simulink model "EV_Modeling_old"  (R2024b)
settings: Solver=FixedStepAuto  StartTime=0.0  StopTime=10382  FixedStep=0.1  RelTol=1e-3
values from neighbouring files (symbols this model uses):
  battery_SOC_SOC = battery_SOC(:,1)    [EV_Truck.m]    (also in simulink.m)
  battery_SOC_voltage = battery_SOC(:,2)    [EV_Truck.m]    (also in simulink.m)
  drag_coefficient_FV1 = table2array(drag_coefficient(:,3))    [simulink.m]
  drag_coefficient_FV2 = table2array(drag_coefficient(:,4))    [simulink.m]
  drag_coefficient_input = table2array(drag_coefficient(:,1))    [simulink.m]
  drag_coefficient_LV = table2array(drag_coefficient(:,2))    [simulink.m]
  electric_consumption_ressistancce = electric_consumption(:,2)    [EV_Truck.m]    (also in simulink.m)
  electric_consumption_voltage = electric_consumption(:,1)    [EV_Truck.m]    (also in simulink.m)
  motor_efficiency_efficiency = table2array(motor_efficiency(2:height(motor_efficiency),2:width(motor_efficiency)))    [EV_Truck.m]    (also in simulink.m)
  motor_efficiency_RPM = table2array(motor_efficiency(2:height(motor_efficiency),1))    [EV_Truck.m]    (also in simulink.m)
  motor_efficiency_torque = transpose(motor_efficiency_torque)    [EV_Truck.m]    (also in simulink.m)
  motor_RPM_torque = table2array(motor_torque(1:14,1))    [EV_Truck.m]    (also in simulink.m)
  motor_torque_RPM = table2array(motor_torque(1:14,2))    [EV_Truck.m]    (also in simulink.m)
undefined symbols (not defined in the file or in its folder): battery_builder_rtmsupport, battery_sli_rtmsupport, C1_mat, C2_mat, c_sqrt, DiscIntNeverNeededParam, dV0_mat, gcbh, n, Wc, Wm, x0
libraries: simulink x87, packLibrary_lib x30, nesl_utility x6, fl_lib x6, simulink_extras x3, mpcadaslib x2, slpidlib x1
(part 8 of 12)

== system EV_Modeling_old/FV1/SOC Estimator (Kalman Filter)1/Kalman Filter/EKF/Delay - X ==
  u : Inport
  SOC0 : Inport  Port=2
  Constant1 : Constant  Value=0  OutDataTypeStr=Inherit: Inherit via back propagation
  Data Type Conversion Inherited : simulink/Signal Attributes/Data Type Conversion Inherited  ConvertRealWorld=Real World Value  DoSatur=off
  Delay : Delay  DelayLength=1  InitialConditionSource=Input port  SampleTime=Ts
      settings: InputPortMap=u0,p4
  Mux : Mux  Inputs=2
  y : Outport
  wires:
  SOC0/1 -> Data Type Conversion Inherited/1, Mux/1
  Mux/1 -> Delay/2
  Delay/1 -> y/1
  u/1 -> Delay/1
  Data Type Conversion Inherited/1 -> Mux/2
  Constant1/1 -> Data Type Conversion Inherited/2

== system EV_Modeling_old/FV1/SOC Estimator (Kalman Filter)1/Kalman Filter/EKF/Jacobian ==
  current : Inport
  Temperature : Inport  Port=2
  x : Inport  Port=3
  -Ts : Gain  Gain=-1
  2-D Lookup Table C1 : Lookup_n-D  NumberOfTableDimensions=1  BreakpointsForDimension1=SOC_vec  BreakpointsForDimension2=T_vec  Table=C1_mat  InternalRulePriority=Speed  RndMeth=Simplest
  2-D Lookup Table R0 : Lookup_n-D  NumberOfTableDimensions=1  BreakpointsForDimension1=SOC_vec  BreakpointsForDimension2=T_vec  Table=R0_mat  InternalRulePriority=Speed  RndMeth=Simplest
  2-D Lookup Table R1 : Lookup_n-D  NumberOfTableDimensions=1  BreakpointsForDimension1=SOC_vec  BreakpointsForDimension2=T_vec  Table=R1_mat  InternalRulePriority=Speed  RndMeth=Simplest
  2-D Lookup Table V0 : Lookup_n-D  NumberOfTableDimensions=1  BreakpointsForDimension1=SOC_vec  BreakpointsForDimension2=T_vec  Table=V0_mat  InternalRulePriority=Speed  RndMeth=Simplest
  2-D Lookup Table dV0 : Lookup_n-D  NumberOfTableDimensions=1  BreakpointsForDimension1=SOC_vec  BreakpointsForDimension2=T_vec  Table=dV0_mat  InternalRulePriority=Speed  RndMeth=Simplest
  Assignment : Assignment  NumberOfDimensions=2  DiagnosticForDimensions=Warning  IndexOptions=Index vector (dialog),Index vector (dialog)  Indices=2,2  OutputSizes=1,1
  Constant : Constant  Value=|  OutDataTypeStr=Inherit: Inherit via back propagation
      | [1 0;
      | 0 0]
  Constant1 : Constant  OutDataTypeStr=Inherit: Inherit via back propagation
  Constant4 : Constant  Value=-1  OutDataTypeStr=Inherit: Inherit via back propagation
  Data Type Conversion Inherited : simulink/Signal Attributes/Data Type Conversion Inherited  ConvertRealWorld=Real World Value  DoSatur=off
  Data Type Conversion Inherited1 : simulink/Signal Attributes/Data Type Conversion Inherited  ConvertRealWorld=Real World Value  DoSatur=off
  Data Type Conversion Inherited2 : simulink/Signal Attributes/Data Type Conversion Inherited  ConvertRealWorld=Real World Value  DoSatur=off
  Gain : Gain  Gain=1/(AH*3600)
  Math Function : Math
  Mux : Mux  Inputs=2
  Mux1 : Mux  Inputs=2
  Probe : Probe  ProbeWidth=off  ProbeComplexSignal=off  ProbeSampleTimeDataType=Same as input
  Product : Product
  Product2 : Product  Inputs=/*
  Product4 : Product
  Product6 : Product
  Selector : Selector  InputPortWidth=2  IndexOptions=Index vector (dialog)  Indices=1  OutputSizes=1
  Selector1 : Selector  InputPortWidth=2  IndexOptions=Index vector (dialog)  Indices=2  OutputSizes=1
  Selector2 : Selector  InputPortWidth=2  IndexOptions=Index vector (dialog)  Indices=1  OutputSizes=1
  Sum : Sum  Inputs=-+|
  Sum2 : Sum  Inputs=+--
  Terminator : Terminator
  Transpose1 : Math  Operator=transpose
  Vt_model : Outport
  H : Outport  Port=2
  F : Outport  Port=3
  G : Outport  Port=4
  wires:
  Gain/1 -> Mux/1
  Selector/1 -> 2-D Lookup Table R1/1, 2-D Lookup Table R0/1, 2-D Lookup Table V0/1, 2-D Lookup Table dV0/1, 2-D Lookup Table C1/1  "SOC"
  x/1 -> Probe/1, Selector/1, Selector1/1
  Math Function/1 -> Sum/1, Assignment/2
  2-D Lookup Table R1/1 -> Product4/2, Product/1  "R1"
  2-D Lookup Table C1/1 -> Product/2  "C1"
  Product2/1 -> Math Function/1
  Assignment/1 -> F/1
  Sum/1 -> Product4/1
  -Ts/1 -> Data Type Conversion Inherited/1, Data Type Conversion Inherited1/1, Gain/1, Product2/2
  Product4/1 -> Mux/2
  Mux/1 -> G/1
  2-D Lookup Table R0/1 -> Product6/1  "R0"
  Product6/1 -> Sum2/2
  Selector1/1 -> Sum2/3  "V1"
  current/1 -> Product6/2
  Mux1/1 -> Transpose1/1
  Transpose1/1 -> H/1
  Sum2/1 -> Vt_model/1
  2-D Lookup Table V0/1 -> Sum2/1  "V0"
  2-D Lookup Table dV0/1 -> Data Type Conversion Inherited2/1, Mux1/1  "dV0"
  Product/1 -> Product2/1  "tau1"
  Probe/1 -> Selector2/1
  Selector2/1 -> -Ts/1
  Data Type Conversion Inherited/1 -> Assignment/1
  Constant/1 -> Data Type Conversion Inherited/2
  Data Type Conversion Inherited1/1 -> Sum/2
  Constant1/1 -> Data Type Conversion Inherited1/2
  Data Type Conversion Inherited2/1 -> Mux1/2
  Constant4/1 -> Data Type Conversion Inherited2/2
  Temperature/1 -> Terminator/1

== system EV_Modeling_old/FV1/SOC Estimator (Kalman Filter)1/Kalman Filter/EKF/Prediction ==
  F : Inport
  G : Inport  Port=2
  xk_k : Inport  Port=3
  Pk_k : Inport  Port=4
  Current : Inport  Port=5
  Constant : Constant  Value=Q  OutDataTypeStr=Inherit: Inherit via back propagation
  Product : Product  Multiplication=Matrix(*)
  Product1 : Product  Multiplication=Matrix(*)
  Product2 : Product  Inputs=3  Multiplication=Matrix(*)
  Sum : Sum  Inputs=|++
  Sum1 : Sum  Inputs=|++
  Transpose : Math  Operator=transpose
  xk1_k : Outport
  Pk1_k : Outport  Port=2
  wires:
  F/1 -> Transpose/1, Product2/1, Product/1
  xk_k/1 -> Product/2
  G/1 -> Product1/1
  Current/1 -> Product1/2
  Product/1 -> Sum/1
  Product1/1 -> Sum/2
  Sum/1 -> xk1_k/1
  Pk_k/1 -> Product2/2
  Transpose/1 -> Product2/3
  Product2/1 -> Sum1/1
  Sum1/1 -> Pk1_k/1
  Constant/1 -> Sum1/2

== system EV_Modeling_old/FV1/SOC Estimator (Kalman Filter)1/Kalman Filter/EKF 2RC/Correction ==
  Vt_error : Inport
  H : Inport  Port=2
  xk1_k : Inport  Port=3
  Pk1_k : Inport  Port=4
  Constant : Constant  Value=R
  Constant1 : Constant  Value=eye(size(R,1))
  Constant2 : Constant  Value=eye(size(Q_2RC,1))
  Data Type Conversion Inherited : simulink/Signal Attributes/Data Type Conversion Inherited  ConvertRealWorld=Real World Value  DoSatur=off
  Data Type Conversion Inherited1 : simulink/Signal Attributes/Data Type Conversion Inherited  ConvertRealWorld=Real World Value  DoSatur=off
  Data Type Conversion Inherited2 : simulink/Signal Attributes/Data Type Conversion Inherited  ConvertRealWorld=Real World Value  DoSatur=off
  Divide : Product  Inputs=*/  Multiplication=Matrix(*)
  Product{,1,3..5} (5 alike) : Product  Multiplication=Matrix(*)
  Product2 : Product  Inputs=3  Multiplication=Matrix(*)
  Sum : Sum  Inputs=++|
  Sum2 : Sum  Inputs=|++
  Sum3 : Sum  Inputs=-+|
  Transpose : Math  Operator=transpose
  xk1_k1 : Outport
  Pk1_k1 : Outport  Port=2
  wires:
  Constant2/1 -> Data Type Conversion Inherited2/2
  Data Type Conversion Inherited2/1 -> Sum3/2
  Constant1/1 -> Data Type Conversion Inherited1/2
  Data Type Conversion Inherited1/1 -> Divide/1
  Constant/1 -> Data Type Conversion Inherited/2
  Data Type Conversion Inherited/1 -> Sum2/2
  H/1 -> Product4/2, Data Type Conversion Inherited2/1, Product2/1, Transpose/1
  Transpose/1 -> Product2/3, Product/2
  Pk1_k/1 -> Product5/2, Product2/2, Product/1
  Product/1 -> Product1/1, Data Type Conversion Inherited1/1
  Product2/1 -> Sum2/1, Data Type Conversion Inherited/1
  Product1/1 -> Product4/1, Product3/1  "Kk1"
  Sum2/1 -> Divide/2
  Divide/1 -> Product1/2
  xk1_k/1 -> Sum/2
  Vt_error/1 -> Product3/2
  Product3/1 -> Sum/1
  Sum/1 -> xk1_k1/1
  Product4/1 -> Sum3/1
  Sum3/1 -> Product5/1
  Product5/1 -> Pk1_k1/1

== system EV_Modeling_old/FV1/SOC Estimator (Kalman Filter)1/Kalman Filter/EKF 2RC/Delay - X ==
  u : Inport
  SOC0 : Inport  Port=2
  Constant1 : Constant  Value=0
  Data Type Conversion Inherited : simulink/Signal Attributes/Data Type Conversion Inherited  ConvertRealWorld=Real World Value  DoSatur=off
  Delay : Delay  DelayLength=1  InitialConditionSource=Input port  SampleTime=Ts
      settings: InputPortMap=u0,p4
  Mux : Mux  Inputs=3
  y : Outport
  wires:
  Constant1/1 -> Data Type Conversion Inherited/2
  Data Type Conversion Inherited/1 -> Mux/3, Mux/2
  SOC0/1 -> Mux/1, Data Type Conversion Inherited/1
  Mux/1 -> Delay/2
  Delay/1 -> y/1
  u/1 -> Delay/1

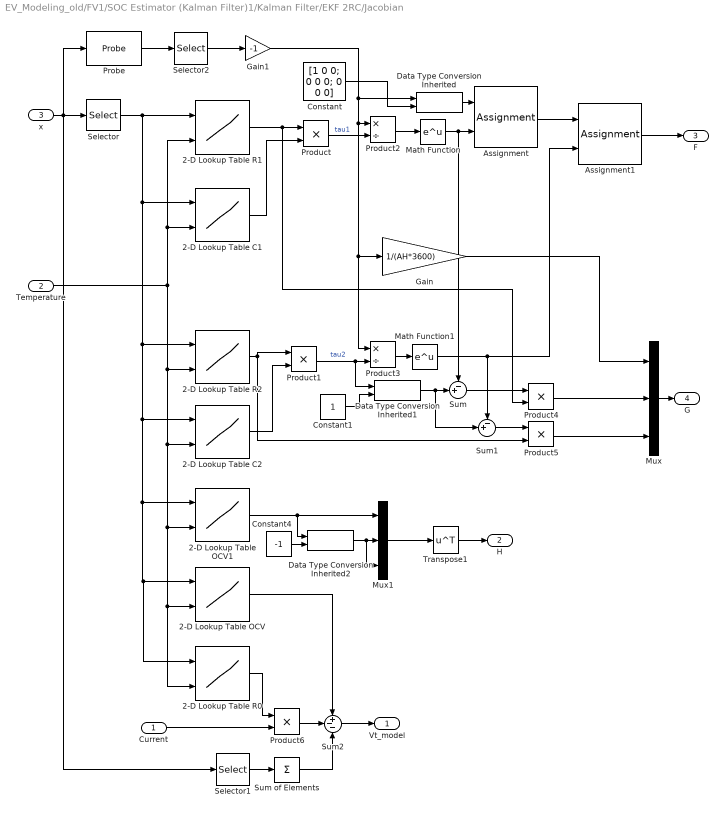
== system EV_Modeling_old/FV1/SOC Estimator (Kalman Filter)1/Kalman Filter/EKF 2RC/Jacobian ==
  Current : Inport
  Temperature : Inport  Port=2
  x : Inport  Port=3
  2-D Lookup Table C1 : Lookup_n-D  BreakpointsForDimension1=SOC_vec  BreakpointsForDimension2=T_vec  Table=C1_mat  InternalRulePriority=Speed  RndMeth=Simplest
      settings: InputPortMap=u0,u1
  2-D Lookup Table C2 : Lookup_n-D  BreakpointsForDimension1=SOC_vec  BreakpointsForDimension2=T_vec  Table=C2_mat  InternalRulePriority=Speed  RndMeth=Simplest
      settings: InputPortMap=u0,u1
  2-D Lookup Table OCV : Lookup_n-D  BreakpointsForDimension1=SOC_vec  BreakpointsForDimension2=T_vec  Table=V0_mat  InternalRulePriority=Speed  RndMeth=Simplest
      settings: InputPortMap=u0,u1
  2-D Lookup Table OCV1 : Lookup_n-D  BreakpointsForDimension1=SOC_vec  BreakpointsForDimension2=T_vec  Table=dV0_mat  InternalRulePriority=Speed  RndMeth=Simplest
      settings: InputPortMap=u0,u1
  2-D Lookup Table R0 : Lookup_n-D  BreakpointsForDimension1=SOC_vec  BreakpointsForDimension2=T_vec  Table=R0_mat  InternalRulePriority=Speed  RndMeth=Simplest
      settings: InputPortMap=u0,u1
  2-D Lookup Table R1 : Lookup_n-D  BreakpointsForDimension1=SOC_vec  BreakpointsForDimension2=T_vec  Table=R1_mat  InternalRulePriority=Speed  RndMeth=Simplest
      settings: InputPortMap=u0,u1
  2-D Lookup Table R2 : Lookup_n-D  BreakpointsForDimension1=SOC_vec  BreakpointsForDimension2=T_vec  Table=R2_mat  InternalRulePriority=Speed  RndMeth=Simplest
      settings: InputPortMap=u0,u1
  Assignment : Assignment  NumberOfDimensions=2  DiagnosticForDimensions=Warning  IndexOptions=Index vector (dialog),Index vector (dialog)  Indices=2,2  OutputSizes=1,1
  Assignment1 : Assignment  NumberOfDimensions=2  DiagnosticForDimensions=Warning  IndexOptions=Index vector (dialog),Index vector (dialog)  Indices=3,3  OutputSizes=1,1
  Constant : Constant  Value=|
      | [1 0  0;
      | 0 0 0;
      | 0 0 0]
  Constant1 : Constant
  Constant4 : Constant  Value=-1
  Data Type Conversion Inherited : simulink/Signal Attributes/Data Type Conversion Inherited  ConvertRealWorld=Real World Value  DoSatur=off
  Data Type Conversion Inherited1 : simulink/Signal Attributes/Data Type Conversion Inherited  ConvertRealWorld=Real World Value  DoSatur=off
  Data Type Conversion Inherited2 : simulink/Signal Attributes/Data Type Conversion Inherited  ConvertRealWorld=Real World Value  DoSatur=off
  Gain : Gain  Gain=1/(AH*3600)
  Gain1 : Gain  Gain=-1
  Math Function : Math
  Math Function1 : Math
  Mux : Mux  Inputs=3
  Mux1 : Mux  Inputs=3
  Probe : Probe  ProbeWidth=off  ProbeComplexSignal=off  ProbeSampleTimeDataType=Same as input
  Product{,1,4..6} (5 alike) : Product
  Product2 : Product  Inputs=*/
  Product3 : Product  Inputs=*/
  Selector : Selector  InputPortWidth=3  IndexOptions=Index vector (dialog)  Indices=1  OutputSizes=1
  Selector1 : Selector  InputPortWidth=3  IndexOptions=Index vector (dialog)  Indices=[2 3]  OutputSizes=1
  Selector2 : Selector  InputPortWidth=2  IndexOptions=Index vector (dialog)  Indices=1  OutputSizes=1
  Sum : Sum  Inputs=-+|
  Sum of Elements : Sum  Inputs=+
  Sum1 : Sum  Inputs=-+|
  Sum2 : Sum  Inputs=+--
  Transpose1 : Math  Operator=transpose
  Vt_model : Outport
  H : Outport  Port=2
  F : Outport  Port=3
  G : Outport  Port=4
  wires:
  Data Type Conversion Inherited2/1 -> Mux1/2, Mux1/3
  Constant4/1 -> Data Type Conversion Inherited2/2
  Constant1/1 -> Data Type Conversion Inherited1/2
  Data Type Conversion Inherited1/1 -> Sum/2, Sum1/2
  Constant/1 -> Data Type Conversion Inherited/2
  Data Type Conversion Inherited/1 -> Assignment/1
  x/1 -> Probe/1, Selector1/1, Selector/1
  Assignment/1 -> Assignment1/1
  Math Function1/1 -> Sum1/1, Assignment1/2
  Math Function/1 -> Assignment/2, Sum/1
  2-D Lookup Table R1/1 -> Product4/2, Product/1
  2-D Lookup Table C1/1 -> Product/2
  2-D Lookup Table R2/1 -> Product1/1, Product5/2
  2-D Lookup Table C2/1 -> Product1/2
  Product/1 -> Product2/2  "tau1"
  Product1/1 -> Product3/2, Data Type Conversion Inherited1/1  "tau2"
  Product2/1 -> Math Function/1
  Product3/1 -> Math Function1/1
  Assignment1/1 -> F/1
  Sum/1 -> Product4/1
  Sum1/1 -> Product5/1
  Gain1/1 -> Product3/1, Gain/1, Product2/1, Data Type Conversion Inherited/1
  Product4/1 -> Mux/2
  Product5/1 -> Mux/3
  Mux/1 -> G/1
  2-D Lookup Table R0/1 -> Product6/1
  Product6/1 -> Sum2/2
  Selector1/1 -> Sum of Elements/1
  Sum of Elements/1 -> Sum2/3
  Current/1 -> Product6/2
  Mux1/1 -> Transpose1/1
  Transpose1/1 -> H/1
  Sum2/1 -> Vt_model/1
  2-D Lookup Table OCV/1 -> Sum2/1
  2-D Lookup Table OCV1/1 -> Mux1/1, Data Type Conversion Inherited2/1
  Temperature/1 -> 2-D Lookup Table R1/2, 2-D Lookup Table C1/2, 2-D Lookup Table R0/2, 2-D Lookup Table OCV/2, 2-D Lookup Table OCV1/2, 2-D Lookup Table C2/2, 2-D Lookup Table R2/2
  Selector/1 -> 2-D Lookup Table R0/1, 2-D Lookup Table OCV/1, 2-D Lookup Table OCV1/1, 2-D Lookup Table C2/1, 2-D Lookup Table R2/1, 2-D Lookup Table C1/1, 2-D Lookup Table R1/1
  Gain/1 -> Mux/1
  Probe/1 -> Selector2/1
  Selector2/1 -> Gain1/1

== system EV_Modeling_old/FV1/SOC Estimator (Kalman Filter)1/Kalman Filter/EKF 2RC/Prediction ==
  F : Inport
  G : Inport  Port=2
  xk_k : Inport  Port=3
  Pk_k : Inport  Port=4
  Current : Inport  Port=5
  Constant : Constant  Value=Q_2RC
  Data Type Conversion Inherited : simulink/Signal Attributes/Data Type Conversion Inherited  ConvertRealWorld=Real World Value  DoSatur=off
  Product : Product  Multiplication=Matrix(*)
  Product1 : Product  Multiplication=Matrix(*)
  Product2 : Product  Inputs=3  Multiplication=Matrix(*)
  Sum : Sum  Inputs=|++
  Sum1 : Sum  Inputs=|++
  Transpose : Math  Operator=transpose
  xk1_k : Outport
  Pk1_k : Outport  Port=2
  wires:
  Constant/1 -> Data Type Conversion Inherited/2
  Data Type Conversion Inherited/1 -> Sum1/2
  F/1 -> Transpose/1, Data Type Conversion Inherited/1, Product2/1, Product/1
  xk_k/1 -> Product/2
  G/1 -> Product1/1
  Current/1 -> Product1/2
  Product/1 -> Sum/1
  Product1/1 -> Sum/2
  Sum/1 -> xk1_k/1
  Pk_k/1 -> Product2/2
  Transpose/1 -> Product2/3
  Product2/1 -> Sum1/1
  Sum1/1 -> Pk1_k/1

== system EV_Modeling_old/FV1/SOC Estimator (Kalman Filter)1/Kalman Filter/UKBF/Prediction-correction ==
  Current : Inport
  Temperature : Inport  Port=2
  Voltage : Inport  Port=3
  X0 : Inport  Port=4
  Integrator1 : Integrator  InitialConditionSource=external
  Measurement function : Subsystem  TreatAsAtomicUnit=on
  State function : Subsystem  TreatAsAtomicUnit=on
  Sum of Elements1 : Sum  Inputs=+  CollapseMode=Specified dimension  CollapseDim=2
  Sum of Elements2 : Sum  Inputs=+  CollapseMode=Specified dimension  CollapseDim=2
  Sum of Elements3 : Sum  Inputs=+  CollapseMode=Specified dimension  CollapseDim=2
  Update A : Subsystem
  Xdot : Subsystem
  xhat : Outport
  wires:
  Integrator1/1 -> State function/3(X), Measurement function/3(X), Xdot/7(X), Update A/1(X)
  Voltage/1 -> Xdot/1(Voltage)
  Measurement function/1(h(X)) -> Xdot/2(h(X))
  State function/1(f(X)) -> Xdot/4(f(X))
  X0/1 -> Integrator1/2
  Current/1 -> State function/1(Current), Measurement function/1(Current)
  Temperature/1 -> State function/2(Temperature), Measurement function/2(Temperature)
  Update A/2(xhat) -> xhat/1
  Update A/1(A(t)) -> Xdot/8(A)
  Xdot/1(Xdot) -> Integrator1/1
  Measurement function/2(h(X)*Wm) -> Sum of Elements1/1
  State function/2(f(X)*Wm) -> Sum of Elements2/1
  State function/3(X*Wm) -> Sum of Elements3/1
  Sum of Elements1/1 -> Xdot/3(mh)
  Sum of Elements2/1 -> Xdot/5(mf)
  Sum of Elements3/1 -> Xdot/6(mx)

== system EV_Modeling_old/FV1/SOC Estimator (Kalman Filter)1/Kalman Filter/UKBF/Sigma points init ==
  x0 : Inport
  A : Inport  Port=2
  Assignment : Assignment  NumberOfDimensions=2  DiagnosticForDimensions=Warning  IndexOptions=Index vector (dialog),Index vector (dialog)  Indices=1:n,1  OutputSizes=1,1
  Assignment1 : Assignment  NumberOfDimensions=2  DiagnosticForDimensions=Warning  IndexOptions=Index vector (dialog),Index vector (dialog)  Indices=1:n,2:n+1  OutputSizes=1,1
  Assignment2 : Assignment  NumberOfDimensions=2  DiagnosticForDimensions=Warning  IndexOptions=Index vector (dialog),Index vector (dialog)  Indices=1:n,n+2:2*n+1  OutputSizes=1,1
  Constant : Constant  Value=zeros(n,2*n+1)
  Constant1 : Constant  Value=ones(1,n)  VectorParams1D=off
  Gain : Gain  Gain=c_sqrt
  Matrix Multiply : Product  Multiplication=Matrix(*)
  Sum : Sum  Inputs=|++
  Sum1 : Sum  Inputs=|+-
  X0 : Outport
  wires:
  A/1 -> Gain/1
  x0/1 -> Matrix Multiply/1, Assignment/2
  Constant1/1 -> Matrix Multiply/2
  Matrix Multiply/1 -> Sum1/1, Sum/1
  Gain/1 -> Sum1/2, Sum/2
  Sum/1 -> Assignment1/2
  Sum1/1 -> Assignment2/2
  Constant/1 -> Assignment/1
  Assignment/1 -> Assignment1/1
  Assignment1/1 -> Assignment2/1
  Assignment2/1 -> X0/1

== system EV_Modeling_old/FV1/SOC Estimator (Kalman Filter)1/Kalman Filter/UKBF 2RC/Prediction-correction ==
  Current : Inport
  Temperature : Inport  Port=2
  Voltage : Inport  Port=3
  X0 : Inport  Port=4
  Integrator1 : Integrator  InitialConditionSource=external
  Measurement function : Subsystem  TreatAsAtomicUnit=on
  State function : Subsystem  TreatAsAtomicUnit=on
  Sum of Elements1 : Sum  Inputs=+  CollapseMode=Specified dimension  CollapseDim=2
  Sum of Elements2 : Sum  Inputs=+  CollapseMode=Specified dimension  CollapseDim=2
  Sum of Elements3 : Sum  Inputs=+  CollapseMode=Specified dimension  CollapseDim=2
  Update A : Subsystem
  Xdot : Subsystem
  xhat : Outport
  wires:
  Integrator1/1 -> State function/3(X), Measurement function/3(X), Xdot/7(X), Update A/1(X)
  Voltage/1 -> Xdot/1(Voltage)
  Measurement function/1(h(X)) -> Xdot/2(h(X))
  State function/1(f(X)) -> Xdot/4(f(X))
  X0/1 -> Integrator1/2
  Current/1 -> State function/1(Current), Measurement function/1(Current)
  Temperature/1 -> State function/2(Temperature), Measurement function/2(Temperature)
  Update A/2(xhat) -> xhat/1
  Update A/1(A(t)) -> Xdot/8(A)
  Xdot/1(Xdot) -> Integrator1/1
  Measurement function/2(h(X)*Wm) -> Sum of Elements1/1
  State function/2(f(X)*Wm) -> Sum of Elements2/1
  State function/3(X*Wm) -> Sum of Elements3/1
  Sum of Elements1/1 -> Xdot/3(mh)
  Sum of Elements2/1 -> Xdot/5(mf)
  Sum of Elements3/1 -> Xdot/6(mx)

== system EV_Modeling_old/FV1/SOC Estimator (Kalman Filter)1/Kalman Filter/UKBF 2RC/Sigma points init ==
  x0 : Inport
  A : Inport  Port=2
  Assignment : Assignment  NumberOfDimensions=2  DiagnosticForDimensions=Warning  IndexOptions=Index vector (dialog),Index vector (dialog)  Indices=1:n,1  OutputSizes=1,1
  Assignment1 : Assignment  NumberOfDimensions=2  DiagnosticForDimensions=Warning  IndexOptions=Index vector (dialog),Index vector (dialog)  Indices=1:n,2:n+1  OutputSizes=1,1
  Assignment2 : Assignment  NumberOfDimensions=2  DiagnosticForDimensions=Warning  IndexOptions=Index vector (dialog),Index vector (dialog)  Indices=1:n,n+2:2*n+1  OutputSizes=1,1
  Constant : Constant  Value=zeros(n,2*n+1)
  Constant1 : Constant  Value=ones(1,n)  VectorParams1D=off
  Gain : Gain  Gain=c_sqrt
  Matrix Multiply : Product  Multiplication=Matrix(*)
  Sum : Sum  Inputs=|++
  Sum1 : Sum  Inputs=|+-
  X0 : Outport
  wires:
  A/1 -> Gain/1
  x0/1 -> Matrix Multiply/1, Assignment/2
  Constant1/1 -> Matrix Multiply/2
  Matrix Multiply/1 -> Sum1/1, Sum/1
  Gain/1 -> Sum1/2, Sum/2
  Sum/1 -> Assignment1/2
  Sum1/1 -> Assignment2/2
  Constant/1 -> Assignment/1
  Assignment/1 -> Assignment1/1
  Assignment1/1 -> Assignment2/1
  Assignment2/1 -> X0/1

== system EV_Modeling_old/FV1/SOC Estimator (Kalman Filter)1/Kalman Filter/UKF/Correction ==
  Vt_error : Inport
  xk1_k : Inport  Port=2
  Pxy : Inport  Port=3
  Py : Inport  Port=4
  Pk1_k : Inport  Port=5
  Math Function : Math  Operator=transpose
  Math Function1 : Math  Operator=transpose
  Product1 : Product  Inputs=*/
  Product3 : Product
  Product5 : Product  Multiplication=Matrix(*)
  Product6 : Product  Inputs=*/
  Sum : Sum  Inputs=++|
  updatePk : MATLAB Function  TreatAsAtomicUnit=on
  xk1_k1 : Outport
  Pk1_k1 : Outport  Port=2
  wires:
  Math Function/1 -> Product5/2
  xk1_k/1 -> Sum/2
  Vt_error/1 -> Product3/2
  Pxy/1 -> Product6/1
  Py/1 -> Math Function1/1, Product6/2, Math Function/1
  Sum/1 -> xk1_k1/1
  Product3/1 -> Sum/1
  Product6/1 -> Product1/1  "Kk1"
  Math Function1/1 -> Product1/2
  Product1/1 -> Product5/1, Product3/1  "Kk1"
  updatePk/1(Pk1_k1) -> Pk1_k1/1
  Product5/1 -> updatePk/1(U)
  Pk1_k/1 -> updatePk/2(Pk1_k)

== system EV_Modeling_old/FV1/SOC Estimator (Kalman Filter)1/Kalman Filter/UKF/Delay - X ==
  u : Inport
  SOC0 : Inport  Port=2
  Constant1 : Constant  Value=0  OutDataTypeStr=Inherit: Inherit via back propagation
  Data Type Conversion Inherited : simulink/Signal Attributes/Data Type Conversion Inherited  ConvertRealWorld=Real World Value  DoSatur=off
  Delay : Delay  DelayLength=1  InitialConditionSource=Input port  SampleTime=Ts
      settings: InputPortMap=u0,p4
  Mux : Mux  Inputs=2
  Reshape : Reshape  OutputDimensionality=Customize  OutputDimensions=[2,1]
  y : Outport
  wires:
  SOC0/1 -> Data Type Conversion Inherited/1, Mux/1
  Mux/1 -> Reshape/1
  Delay/1 -> y/1
  u/1 -> Delay/1
  Reshape/1 -> Delay/2
  Data Type Conversion Inherited/1 -> Mux/2
  Constant1/1 -> Data Type Conversion Inherited/2

== system EV_Modeling_old/FV1/SOC Estimator (Kalman Filter)1/Kalman Filter/UKF/Prediction ==
  Current : Inport
  Temperature : Inport  Port=2
  X : Inport  Port=3
  Constant : Constant  Value=diag(Wc)  OutDataTypeStr=Inherit: Inherit via back propagation
  Data Type Conversion Inherited : simulink/Signal Attributes/Data Type Conversion Inherited  ConvertRealWorld=Real World Value  DoSatur=off
  Math Function : Math  Operator=transpose
  Measurement function : Subsystem  TreatAsAtomicUnit=on
  Product1 : Product  Multiplication=Matrix(*)
  Product5 : Product  Multiplication=Matrix(*)
  State function : Subsystem  TreatAsAtomicUnit=on
  Sum of Elements : Sum  Inputs=+  CollapseMode=Specified dimension  CollapseDim=2
  Sum of Elements1 : Sum  Inputs=+  CollapseMode=Specified dimension  CollapseDim=2
  updatePx : MATLAB Function  TreatAsAtomicUnit=on
  updatePy : MATLAB Function  TreatAsAtomicUnit=on
  Yk1_k : Outport
  Xk1_k : Outport  Port=2
  Pxy : Outport  Port=3
  Py : Outport  Port=4
  Pk1k : Outport  Port=5
  wires:
  Current/1 -> Measurement function/1(Current), State function/1(Current)
  X/1 -> State function/3(X)
  Temperature/1 -> Measurement function/2(Temperature), State function/2(Temperature)
  State function/2(Wm_i*xk1_i) -> Sum of Elements/1
  State function/1(xk1) -> updatePx/1(X), Measurement function/3(X)
  Measurement function/2(Wm_i*y_i) -> Sum of Elements1/1
  Sum of Elements1/1 -> updatePy/2(y), Yk1_k/1
  Sum of Elements/1 -> updatePx/2(x), Xk1_k/1
  Measurement function/1(y) -> updatePy/1(Y)
  updatePx/2(X1) -> Data Type Conversion Inherited/1, Product5/1
  updatePy/2(Y1) -> Math Function/1
  Product5/1 -> Product1/1
  Math Function/1 -> Product1/2
  Product1/1 -> Pxy/1
  updatePy/1(Py) -> Py/1
  updatePx/1(Pk1k) -> Pk1k/1
  Data Type Conversion Inherited/1 -> Product5/2
  Constant/1 -> Data Type Conversion Inherited/2

== system EV_Modeling_old/FV1/SOC Estimator (Kalman Filter)1/Kalman Filter/UKF/Sigma points ==
  x : Inport
  P : Inport  Port=2
  Assignment : Assignment  NumberOfDimensions=2  DiagnosticForDimensions=Warning  IndexOptions=Index vector (dialog),Index vector (dialog)  Indices=1:n,1  OutputSizes=1,1
  Assignment1 : Assignment  NumberOfDimensions=2  DiagnosticForDimensions=Warning  IndexOptions=Index vector (dialog),Index vector (dialog)  Indices=1:n,2:n+1  OutputSizes=1,1
  Assignment2 : Assignment  NumberOfDimensions=2  DiagnosticForDimensions=Warning  IndexOptions=Index vector (dialog),Index vector (dialog)  Indices=1:n,n+2:2*n+1  OutputSizes=1,1
  Constant : Constant  Value=zeros(n,2*n+1)  OutDataTypeStr=Inherit: Inherit via back propagation
  Constant1 : Constant  Value=ones(1,n)  VectorParams1D=off  OutDataTypeStr=Inherit: Inherit via back propagation
  Data Type Conversion Inherited : simulink/Signal Attributes/Data Type Conversion Inherited  ConvertRealWorld=Real World Value  DoSatur=off
  Data Type Conversion Inherited1 : simulink/Signal Attributes/Data Type Conversion Inherited  ConvertRealWorld=Real World Value  DoSatur=off
  Gain : Gain  Gain=c_sqrt
  Matrix Multiply : Product  Multiplication=Matrix(*)
  Sum : Sum  Inputs=|++
  Sum1 : Sum  Inputs=|+-
  X : Outport
  wires:
  P/1 -> Gain/1
  x/1 -> Matrix Multiply/1, Data Type Conversion Inherited/1, Assignment/2, Data Type Conversion Inherited1/1
  Matrix Multiply/1 -> Sum1/1, Sum/1
  Gain/1 -> Sum1/2, Sum/2
  Sum/1 -> Assignment1/2
  Sum1/1 -> Assignment2/2
  Assignment/1 -> Assignment1/1
  Assignment1/1 -> Assignment2/1
  Assignment2/1 -> X/1
  Data Type Conversion Inherited/1 -> Assignment/1
  Constant/1 -> Data Type Conversion Inherited/2
  Data Type Conversion Inherited1/1 -> Matrix Multiply/2
  Constant1/1 -> Data Type Conversion Inherited1/2

== system EV_Modeling_old/FV1/SOC Estimator (Kalman Filter)1/Kalman Filter/UKF 2RC/Correction ==
  Vt_error : Inport
  xk1_k : Inport  Port=2
  Pxy : Inport  Port=3
  Py : Inport  Port=4
  Pk1_k : Inport  Port=5
  Math Function : Math  Operator=transpose
  Math Function1 : Math  Operator=transpose
  Product1 : Product  Inputs=*/
  Product3 : Product
  Product5 : Product  Multiplication=Matrix(*)
  Product6 : Product  Inputs=*/
  Sum : Sum  Inputs=++|
  updatePk : MATLAB Function  TreatAsAtomicUnit=on
  xk1_k1 : Outport
  Pk1_k1 : Outport  Port=2
  wires:
  Math Function/1 -> Product5/2
  xk1_k/1 -> Sum/2
  Vt_error/1 -> Product3/2
  Pxy/1 -> Product6/1
  Py/1 -> Math Function1/1, Product6/2, Math Function/1
  Sum/1 -> xk1_k1/1
  Product3/1 -> Sum/1
  Product6/1 -> Product1/1  "Kk1"
  Math Function1/1 -> Product1/2
  Product1/1 -> Product5/1, Product3/1  "Kk1"
  updatePk/1(Pk1_k1) -> Pk1_k1/1
  Product5/1 -> updatePk/1(U)
  Pk1_k/1 -> updatePk/2(Pk1_k)

== system EV_Modeling_old/FV1/SOC Estimator (Kalman Filter)1/Kalman Filter/UKF 2RC/Delay - X ==
  u : Inport
  SOC0 : Inport  Port=2
  Constant1 : Constant  Value=0  OutDataTypeStr=Inherit: Inherit via back propagation
  Data Type Conversion Inherited : simulink/Signal Attributes/Data Type Conversion Inherited  ConvertRealWorld=Real World Value  DoSatur=off
  Delay : Delay  DelayLength=1  InitialConditionSource=Input port  SampleTime=Ts
      settings: InputPortMap=u0,p4
  Mux : Mux  Inputs=3
  Reshape : Reshape  OutputDimensionality=Customize  OutputDimensions=[n,1]
  y : Outport
  wires:
  SOC0/1 -> Data Type Conversion Inherited/1, Mux/1
  Mux/1 -> Reshape/1
  Delay/1 -> y/1
  u/1 -> Delay/1
  Reshape/1 -> Delay/2
  Data Type Conversion Inherited/1 -> Mux/2, Mux/3
  Constant1/1 -> Data Type Conversion Inherited/2

== system EV_Modeling_old/FV1/SOC Estimator (Kalman Filter)1/Kalman Filter/UKF 2RC/Prediction ==
  Current : Inport
  Temperature : Inport  Port=2
  X : Inport  Port=3
  Constant : Constant  Value=diag(Wc)  OutDataTypeStr=Inherit: Inherit via back propagation
  Data Type Conversion Inherited : simulink/Signal Attributes/Data Type Conversion Inherited  ConvertRealWorld=Real World Value  DoSatur=off
  Math Function : Math  Operator=transpose
  Measurement function : Subsystem  TreatAsAtomicUnit=on
  Product1 : Product  Multiplication=Matrix(*)
  Product5 : Product  Multiplication=Matrix(*)
  State function : Subsystem  TreatAsAtomicUnit=on
  Sum of Elements : Sum  Inputs=+  CollapseMode=Specified dimension  CollapseDim=2
  Sum of Elements1 : Sum  Inputs=+  CollapseMode=Specified dimension  CollapseDim=2
  updatePx : MATLAB Function  TreatAsAtomicUnit=on
  updatePy : MATLAB Function  TreatAsAtomicUnit=on
  Yk1_k : Outport
  Xk1_k : Outport  Port=2
  Pxy : Outport  Port=3
  Py : Outport  Port=4
  Pk1k : Outport  Port=5
  wires:
  Current/1 -> Measurement function/1(Current), State function/1(Current)
  X/1 -> State function/3(X)
  Temperature/1 -> Measurement function/2(Temperature), State function/2(Temperature)
  State function/2(Wm_i*xk1_i) -> Sum of Elements/1
  State function/1(xk1) -> updatePx/1(X), Measurement function/3(X)
  Measurement function/2(Wm_i*y_i) -> Sum of Elements1/1
  Sum of Elements1/1 -> updatePy/2(y), Yk1_k/1
  Sum of Elements/1 -> updatePx/2(x), Xk1_k/1
  Measurement function/1(y) -> updatePy/1(Y)
  updatePx/2(X1) -> Data Type Conversion Inherited/1, Product5/1
  updatePy/2(Y1) -> Math Function/1
  Product5/1 -> Product1/1
  Math Function/1 -> Product1/2
  Product1/1 -> Pxy/1
  updatePy/1(Py) -> Py/1
  updatePx/1(Pk1k) -> Pk1k/1
  Data Type Conversion Inherited/1 -> Product5/2
  Constant/1 -> Data Type Conversion Inherited/2

== system EV_Modeling_old/FV1/SOC Estimator (Kalman Filter)1/Kalman Filter/UKF 2RC/Sigma points ==
  x : Inport
  P : Inport  Port=2
  Assignment : Assignment  NumberOfDimensions=2  DiagnosticForDimensions=Warning  IndexOptions=Index vector (dialog),Index vector (dialog)  Indices=1:n,1  OutputSizes=1,1
  Assignment1 : Assignment  NumberOfDimensions=2  DiagnosticForDimensions=Warning  IndexOptions=Index vector (dialog),Index vector (dialog)  Indices=1:n,2:n+1  OutputSizes=1,1
  Assignment2 : Assignment  NumberOfDimensions=2  DiagnosticForDimensions=Warning  IndexOptions=Index vector (dialog),Index vector (dialog)  Indices=1:n,n+2:2*n+1  OutputSizes=1,1
  Constant : Constant  Value=zeros(n,2*n+1)  OutDataTypeStr=Inherit: Inherit via back propagation
  Constant1 : Constant  Value=ones(1,n)  VectorParams1D=off  OutDataTypeStr=Inherit: Inherit via back propagation
  Data Type Conversion Inherited : simulink/Signal Attributes/Data Type Conversion Inherited  ConvertRealWorld=Real World Value  DoSatur=off
  Data Type Conversion Inherited1 : simulink/Signal Attributes/Data Type Conversion Inherited  ConvertRealWorld=Real World Value  DoSatur=off
  Gain : Gain  Gain=c_sqrt
  Matrix Multiply : Product  Multiplication=Matrix(*)
  Sum : Sum  Inputs=|++
  Sum1 : Sum  Inputs=|+-
  X : Outport
  wires:
  P/1 -> Gain/1
  x/1 -> Matrix Multiply/1, Data Type Conversion Inherited/1, Assignment/2, Data Type Conversion Inherited1/1
  Matrix Multiply/1 -> Sum1/1, Sum/1
  Gain/1 -> Sum1/2, Sum/2
  Sum/1 -> Assignment1/2
  Sum1/1 -> Assignment2/2
  Assignment/1 -> Assignment1/1
  Assignment1/1 -> Assignment2/1
  Assignment2/1 -> X/1
  Data Type Conversion Inherited/1 -> Assignment/1
  Constant/1 -> Data Type Conversion Inherited/2
  Data Type Conversion Inherited1/1 -> Matrix Multiply/2
  Constant1/1 -> Data Type Conversion Inherited1/2

== system EV_Modeling_old/FV2/SOC Estimator (Kalman Filter)1/Kalman Filter/EKBF/Jacobian ==
  current : Inport
  Temperature : Inport  Port=2
  x : Inport  Port=3
  2-D Lookup Table C1 : Lookup_n-D  BreakpointsForDimension1=SOC_vec  BreakpointsForDimension2=T_vec  Table=C1_mat  InternalRulePriority=Speed  RndMeth=Simplest
      settings: InputPortMap=u0,u1
  2-D Lookup Table R0 : Lookup_n-D  BreakpointsForDimension1=SOC_vec  BreakpointsForDimension2=T_vec  Table=R0_mat  InternalRulePriority=Speed  RndMeth=Simplest
      settings: InputPortMap=u0,u1
  2-D Lookup Table R1 : Lookup_n-D  BreakpointsForDimension1=SOC_vec  BreakpointsForDimension2=T_vec  Table=R1_mat  InternalRulePriority=Speed  RndMeth=Simplest
      settings: InputPortMap=u0,u1
  2-D Lookup Table V0 : Lookup_n-D  BreakpointsForDimension1=SOC_vec  BreakpointsForDimension2=T_vec  Table=V0_mat  InternalRulePriority=Speed  RndMeth=Simplest
      settings: InputPortMap=u0,u1
  2-D Lookup Table dV0 : Lookup_n-D  BreakpointsForDimension1=SOC_vec  BreakpointsForDimension2=T_vec  Table=dV0_mat  InternalRulePriority=Speed  RndMeth=Simplest
      settings: InputPortMap=u0,u1
  Add1 : Sum  Inputs=-+
  Assignment : Assignment  NumberOfDimensions=2  DiagnosticForDimensions=Warning  IndexOptions=Index vector (dialog),Index vector (dialog)  Indices=2,2  OutputSizes=1,1
  Constant : Constant  Value=|
      | [0 0;
      | 0 0]
  Constant3 : Constant  Value=-1
  Constant4 : Constant  Value=-1
  Divide1 : Product  Inputs=*/
  Divide2 : Product  Inputs=/*
  Gain : Gain  Gain=-1/(AH*3600)
  Mux : Mux  Inputs=2
  Mux1 : Mux  Inputs=2
  Product : Product
  Product2 : Product  Inputs=/*
  Product6 : Product
  Selector : Selector  InputPortWidth=2  IndexOptions=Index vector (dialog)  Indices=1  OutputSizes=1
  Selector1 : Selector  InputPortWidth=2  IndexOptions=Index vector (dialog)  Indices=2  OutputSizes=1
  Sum2 : Sum  Inputs=+--
  Transpose1 : Math  Operator=transpose
  Vt_model : Outport
  f(x) : Outport  Port=2
  F : Outport  Port=3
  H : Outport  Port=4
  wires:
  Product/1 -> Product2/1, Divide2/1  "tau1"
  2-D Lookup Table V0/1 -> Sum2/1  "V0"
  Sum2/1 -> Vt_model/1
  Selector1/1 -> Sum2/3, Divide2/2  "V1"
  Product6/1 -> Sum2/2
  2-D Lookup Table R0/1 -> Product6/1  "R0"
  Constant3/1 -> Product2/2
  Assignment/1 -> F/1
  Product2/1 -> Assignment/2
  Constant/1 -> Assignment/1
  Selector/1 -> 2-D Lookup Table C1/1, 2-D Lookup Table dV0/1, 2-D Lookup Table V0/1, 2-D Lookup Table R0/1, 2-D Lookup Table R1/1  "SOC"
  Temperature/1 -> 2-D Lookup Table dV0/2, 2-D Lookup Table V0/2, 2-D Lookup Table R0/2, 2-D Lookup Table C1/2, 2-D Lookup Table R1/2
  x/1 -> Selector1/1, Selector/1
  Mux1/1 -> Transpose1/1
  Transpose1/1 -> H/1
  Constant4/1 -> Mux1/2
  2-D Lookup Table dV0/1 -> Mux1/1  "dV0"
  Divide1/1 -> Add1/2  "Current/C1"
  Mux/1 -> f(x)/1
  2-D Lookup Table C1/1 -> Divide1/2, Product/2  "C1"
  2-D Lookup Table R1/1 -> Product/1  "R1"
  Add1/1 -> Mux/2
  current/1 -> Product6/2, Gain/1, Divide1/1  "Current"
  Gain/1 -> Mux/1
  Divide2/1 -> Add1/1

== system EV_Modeling_old/FV2/SOC Estimator (Kalman Filter)1/Kalman Filter/EKBF/Prediction-correction ==
  f(x) : Inport
  F : Inport  Port=2
  H : Inport  Port=3
  InitialSOC : Inport  Port=4
  Vt_error : Inport  Port=5
  Constant : Constant  Value=Q
  Constant1 : Constant  Value=double(R)
  Constant2 : Constant  Value=eye(size(R,1))
  Constant3 : Constant  Value=0
  Divide : Product  Inputs=*/  Multiplication=Matrix(*)
  Integrator : Integrator  InitialCondition=double(P0)
  Integrator1 : Integrator  InitialConditionSource=external  InitialCondition=x0
  Mux : Mux  Inputs=2
  Product : Product  Multiplication=Matrix(*)
  Product3 : Product  Multiplication=Matrix(*)
  Product4 : Product  Inputs=3  Multiplication=Matrix(*)
  Product5 : Product  Inputs=3  Multiplication=Matrix(*)
  Product6 : Product  Multiplication=Matrix(*)
  Reshape : Reshape  OutputDimensionality=Customize  OutputDimensions=[n,1]
  Sum : Sum  Inputs=++-+
  Sum2 : Sum  Inputs=|++
  Transpose : Math  Operator=transpose
  Transpose1 : Math  Operator=transpose
  x : Outport
  wires:
  f(x)/1 -> Sum2/1
  Sum2/1 -> Integrator1/1
  Product6/1 -> Sum2/2
  Vt_error/1 -> Product6/2
  H/1 -> Product4/2, Transpose1/1
  F/1 -> Transpose/1, Product/1
  Integrator1/1 -> x/1
  Product5/1 -> Product6/1, Product4/1
  Constant2/1 -> Divide/1
  Divide/1 -> Product5/3
  Constant1/1 -> Divide/2
  Transpose1/1 -> Product5/2
  Sum/1 -> Integrator/1  "Pdot"
  Constant/1 -> Sum/4
  Product4/1 -> Sum/3
  Transpose/1 -> Product3/2
  Product3/1 -> Sum/2
  Product/1 -> Sum/1
  Integrator/1 -> Product5/1, Product4/3, Product/2, Product3/1
  Mux/1 -> Reshape/1
  InitialSOC/1 -> Mux/1
  Constant3/1 -> Mux/2
  Reshape/1 -> Integrator1/2

== system EV_Modeling_old/FV2/SOC Estimator (Kalman Filter)1/Kalman Filter/EKBF 2RC/Jacobian ==
  current : Inport
  Temperature : Inport  Port=2
  x : Inport  Port=3
  2-D Lookup Table C1 : Lookup_n-D  BreakpointsForDimension1=SOC_vec  BreakpointsForDimension2=T_vec  Table=C1_mat  InternalRulePriority=Speed  RndMeth=Simplest
      settings: InputPortMap=u0,u1
  2-D Lookup Table C2 : Lookup_n-D  BreakpointsForDimension1=SOC_vec  BreakpointsForDimension2=T_vec  Table=C2_mat  InternalRulePriority=Speed  RndMeth=Simplest
      settings: InputPortMap=u0,u1
  2-D Lookup Table R0 : Lookup_n-D  BreakpointsForDimension1=SOC_vec  BreakpointsForDimension2=T_vec  Table=R0_mat  InternalRulePriority=Speed  RndMeth=Simplest
      settings: InputPortMap=u0,u1
  2-D Lookup Table R1 : Lookup_n-D  BreakpointsForDimension1=SOC_vec  BreakpointsForDimension2=T_vec  Table=R1_mat  InternalRulePriority=Speed  RndMeth=Simplest
      settings: InputPortMap=u0,u1
  2-D Lookup Table R2 : Lookup_n-D  BreakpointsForDimension1=SOC_vec  BreakpointsForDimension2=T_vec  Table=R2_mat  InternalRulePriority=Speed  RndMeth=Simplest
      settings: InputPortMap=u0,u1
  2-D Lookup Table V0 : Lookup_n-D  BreakpointsForDimension1=SOC_vec  BreakpointsForDimension2=T_vec  Table=V0_mat  InternalRulePriority=Speed  RndMeth=Simplest
      settings: InputPortMap=u0,u1
  2-D Lookup Table dV0 : Lookup_n-D  BreakpointsForDimension1=SOC_vec  BreakpointsForDimension2=T_vec  Table=dV0_mat  InternalRulePriority=Speed  RndMeth=Simplest
      settings: InputPortMap=u0,u1
  Add1 : Sum  Inputs=-+
  Add2 : Sum  Inputs=-+
  Assignment : Assignment  NumberOfDimensions=2  DiagnosticForDimensions=Warning  IndexOptions=Index vector (dialog),Index vector (dialog)  Indices=2,2  OutputSizes=1,1
  Assignment1 : Assignment  NumberOfDimensions=2  DiagnosticForDimensions=Warning  IndexOptions=Index vector (dialog),Index vector (dialog)  Indices=3,3  OutputSizes=1,1
  Constant : Constant  Value=|
      | [0 0 0;
      | 0 0 0;0 0 0]
  Constant3 : Constant  Value=-1
  Constant4 : Constant  Value=-1
  Divide1 : Product  Inputs=*/
  Divide2 : Product  Inputs=/*
  Divide3 : Product  Inputs=/*
  Divide4 : Product  Inputs=*/
  Gain : Gain  Gain=-1/(AH*3600)
  Mux : Mux  Inputs=3
  Mux1 : Mux  Inputs=3
  Product : Product
  Product2 : Product  Inputs=/*
  Product3 : Product
  Product4 : Product  Inputs=*/
  Product6 : Product
  Selector : Selector  InputPortWidth=3  IndexOptions=Index vector (dialog)  Indices=1  OutputSizes=1
  Selector2 : Selector  InputPortWidth=3  IndexOptions=Index vector (dialog)  Indices=2  OutputSizes=1
  Selector3 : Selector  InputPortWidth=3  IndexOptions=Index vector (dialog)  Indices=3  OutputSizes=1
  Sum : Sum
  Sum2 : Sum  Inputs=+--
  Transpose1 : Math  Operator=transpose
  Vt_model : Outport
  f(x) : Outport  Port=2
  F : Outport  Port=3
  H : Outport  Port=4
  wires:
  Divide4/1 -> Add2/2  "Current/C2"
  Add2/1 -> Mux/3
  Divide3/1 -> Add2/1
  Selector3/1 -> Sum/2, Divide3/2  "V2"
  Selector2/1 -> Sum/1, Divide2/2  "V1"
  Sum/1 -> Sum2/3  "V1+V2"
  Product4/1 -> Assignment1/2
  Product3/1 -> Product4/2, Divide3/1  "tau2"
  2-D Lookup Table C2/1 -> Divide4/2, Product3/2
  2-D Lookup Table R2/1 -> Product3/1
  Assignment1/1 -> F/1
  Assignment/1 -> Assignment1/1
  Product/1 -> Product2/1, Divide2/1  "tau1"
  2-D Lookup Table V0/1 -> Sum2/1  "V0"
  Sum2/1 -> Vt_model/1
  Product6/1 -> Sum2/2
  2-D Lookup Table R0/1 -> Product6/1  "R0"
  Constant3/1 -> Product4/1, Product2/2
  Product2/1 -> Assignment/2
  Constant/1 -> Assignment/1
  Selector/1 -> 2-D Lookup Table C1/1, 2-D Lookup Table dV0/1, 2-D Lookup Table V0/1, 2-D Lookup Table R0/1, 2-D Lookup Table C2/1, 2-D Lookup Table R2/1, 2-D Lookup Table R1/1  "SOC"
  Temperature/1 -> 2-D Lookup Table dV0/2, 2-D Lookup Table V0/2, 2-D Lookup Table R0/2, 2-D Lookup Table C2/2, 2-D Lookup Table R2/2, 2-D Lookup Table C1/2, 2-D Lookup Table R1/2
  x/1 -> Selector2/1, Selector3/1, Selector/1
  Mux1/1 -> Transpose1/1
  Transpose1/1 -> H/1
  Constant4/1 -> Mux1/2, Mux1/3
  2-D Lookup Table dV0/1 -> Mux1/1  "dV0"
  Divide1/1 -> Add1/2  "Current/C1"
  Mux/1 -> f(x)/1
  2-D Lookup Table C1/1 -> Divide1/2, Product/2  "C1"
  2-D Lookup Table R1/1 -> Product/1  "R1"
  Add1/1 -> Mux/2
  current/1 -> Product6/2, Gain/1, Divide1/1, Divide4/1  "Current"
  Gain/1 -> Mux/1
  Divide2/1 -> Add1/1

== system EV_Modeling_old/FV2/SOC Estimator (Kalman Filter)1/Kalman Filter/EKBF 2RC/Prediction-correction ==
  f(x) : Inport
  F : Inport  Port=2
  H : Inport  Port=3
  InitialSOC : Inport  Port=4
  Vt_error : Inport  Port=5
  Constant : Constant  Value=Q_2RC
  Constant1 : Constant  Value=double(R)
  Constant2 : Constant  Value=eye(size(R,1))
  Constant3 : Constant  Value=0
  Divide : Product  Inputs=*/  Multiplication=Matrix(*)
  Integrator : Integrator  InitialCondition=double(P0_2RC)
  Integrator1 : Integrator  InitialConditionSource=external  InitialCondition=x0
  Mux : Mux  Inputs=3
  Product : Product  Multiplication=Matrix(*)
  Product3 : Product  Multiplication=Matrix(*)
  Product4 : Product  Inputs=3  Multiplication=Matrix(*)
  Product5 : Product  Inputs=3  Multiplication=Matrix(*)
  Product6 : Product  Multiplication=Matrix(*)
  Sum : Sum  Inputs=++-+
  Sum2 : Sum  Inputs=|++
  Transpose : Math  Operator=transpose
  Transpose1 : Math  Operator=transpose
  x : Outport
  wires:
  Constant3/1 -> Mux/2, Mux/3
  Constant2/1 -> Divide/1
  Constant1/1 -> Divide/2
  Constant/1 -> Sum/4
  InitialSOC/1 -> Mux/1
  Mux/1 -> Integrator1/2
  Integrator/1 -> Product3/1, Product/2, Product4/3, Product5/1
  Product/1 -> Sum/1
  Product3/1 -> Sum/2
  Transpose/1 -> Product3/2
  Product4/1 -> Sum/3
  Sum/1 -> Integrator/1  "Pdot"
  Transpose1/1 -> Product5/2
  Divide/1 -> Product5/3
  Product5/1 -> Product4/1, Product6/1
  Integrator1/1 -> x/1
  F/1 -> Product/1, Transpose/1
  H/1 -> Transpose1/1, Product4/2
  Vt_error/1 -> Product6/2
  Product6/1 -> Sum2/2
  Sum2/1 -> Integrator1/1
  f(x)/1 -> Sum2/1

== system EV_Modeling_old/FV2/SOC Estimator (Kalman Filter)1/Kalman Filter/EKF/Correction ==
  Vt_error : Inport
  H : Inport  Port=2
  xk1_k : Inport  Port=3
  Pk1_k : Inport  Port=4
  Constant : Constant  Value=R
  Constant1 : Constant  Value=eye(size(R,1))
  Constant2 : Constant  Value=eye(size(Q,1))  OutDataTypeStr=Inherit: Inherit via back propagation
  Data Type Conversion Inherited : simulink/Signal Attributes/Data Type Conversion Inherited  ConvertRealWorld=Real World Value  DoSatur=off
  Data Type Conversion Inherited1 : simulink/Signal Attributes/Data Type Conversion Inherited  ConvertRealWorld=Real World Value  DoSatur=off
  Divide : Product  Inputs=*/  Multiplication=Matrix(*)
  Product{,1,3..5} (5 alike) : Product  Multiplication=Matrix(*)
  Product2 : Product  Inputs=3  Multiplication=Matrix(*)
  Sum : Sum  Inputs=++|
  Sum2 : Sum  Inputs=|++
  Sum3 : Sum  Inputs=-+|
  Transpose : Math  Operator=transpose
  xk1_k1 : Outport
  Pk1_k1 : Outport  Port=2
  wires:
  H/1 -> Product4/2, Product2/1, Transpose/1
  Transpose/1 -> Product2/3, Product/2
  Pk1_k/1 -> Product5/2, Product2/2, Product/1
  Product/1 -> Data Type Conversion Inherited1/1, Product1/1
  Product2/1 -> Sum2/1
  Constant/1 -> Sum2/2
  Product1/1 -> Product4/1, Product3/1  "Kk1"
  Sum2/1 -> Divide/2
  Divide/1 -> Product1/2
  xk1_k/1 -> Sum/2
  Vt_error/1 -> Product3/2
  Product3/1 -> Sum/1
  Sum/1 -> xk1_k1/1
  Product4/1 -> Data Type Conversion Inherited/1, Sum3/1
  Sum3/1 -> Product5/1
  Product5/1 -> Pk1_k1/1
  Data Type Conversion Inherited/1 -> Sum3/2
  Constant2/1 -> Data Type Conversion Inherited/2
  Data Type Conversion Inherited1/1 -> Divide/1
  Constant1/1 -> Data Type Conversion Inherited1/2

== system EV_Modeling_old/FV2/SOC Estimator (Kalman Filter)1/Kalman Filter/EKF/Delay - X ==
  u : Inport
  SOC0 : Inport  Port=2
  Constant1 : Constant  Value=0  OutDataTypeStr=Inherit: Inherit via back propagation
  Data Type Conversion Inherited : simulink/Signal Attributes/Data Type Conversion Inherited  ConvertRealWorld=Real World Value  DoSatur=off
  Delay : Delay  DelayLength=1  InitialConditionSource=Input port  SampleTime=Ts
      settings: InputPortMap=u0,p4
  Mux : Mux  Inputs=2
  y : Outport
  wires:
  SOC0/1 -> Data Type Conversion Inherited/1, Mux/1
  Mux/1 -> Delay/2
  Delay/1 -> y/1
  u/1 -> Delay/1
  Data Type Conversion Inherited/1 -> Mux/2
  Constant1/1 -> Data Type Conversion Inherited/2

== system EV_Modeling_old/FV2/SOC Estimator (Kalman Filter)1/Kalman Filter/EKF/Jacobian ==
  current : Inport
  Temperature : Inport  Port=2
  x : Inport  Port=3
  -Ts : Gain  Gain=-1
  2-D Lookup Table C1 : Lookup_n-D  NumberOfTableDimensions=1  BreakpointsForDimension1=SOC_vec  BreakpointsForDimension2=T_vec  Table=C1_mat  InternalRulePriority=Speed  RndMeth=Simplest
  2-D Lookup Table R0 : Lookup_n-D  NumberOfTableDimensions=1  BreakpointsForDimension1=SOC_vec  BreakpointsForDimension2=T_vec  Table=R0_mat  InternalRulePriority=Speed  RndMeth=Simplest
  2-D Lookup Table R1 : Lookup_n-D  NumberOfTableDimensions=1  BreakpointsForDimension1=SOC_vec  BreakpointsForDimension2=T_vec  Table=R1_mat  InternalRulePriority=Speed  RndMeth=Simplest
  2-D Lookup Table V0 : Lookup_n-D  NumberOfTableDimensions=1  BreakpointsForDimension1=SOC_vec  BreakpointsForDimension2=T_vec  Table=V0_mat  InternalRulePriority=Speed  RndMeth=Simplest
  2-D Lookup Table dV0 : Lookup_n-D  NumberOfTableDimensions=1  BreakpointsForDimension1=SOC_vec  BreakpointsForDimension2=T_vec  Table=dV0_mat  InternalRulePriority=Speed  RndMeth=Simplest
  Assignment : Assignment  NumberOfDimensions=2  DiagnosticForDimensions=Warning  IndexOptions=Index vector (dialog),Index vector (dialog)  Indices=2,2  OutputSizes=1,1
  Constant : Constant  Value=|  OutDataTypeStr=Inherit: Inherit via back propagation
      | [1 0;
      | 0 0]
  Constant1 : Constant  OutDataTypeStr=Inherit: Inherit via back propagation
  Constant4 : Constant  Value=-1  OutDataTypeStr=Inherit: Inherit via back propagation
  Data Type Conversion Inherited : simulink/Signal Attributes/Data Type Conversion Inherited  ConvertRealWorld=Real World Value  DoSatur=off
  Data Type Conversion Inherited1 : simulink/Signal Attributes/Data Type Conversion Inherited  ConvertRealWorld=Real World Value  DoSatur=off
  Data Type Conversion Inherited2 : simulink/Signal Attributes/Data Type Conversion Inherited  ConvertRealWorld=Real World Value  DoSatur=off
  Gain : Gain  Gain=1/(AH*3600)
  Math Function : Math
  Mux : Mux  Inputs=2
  Mux1 : Mux  Inputs=2
  Probe : Probe  ProbeWidth=off  ProbeComplexSignal=off  ProbeSampleTimeDataType=Same as input
  Product : Product
  Product2 : Product  Inputs=/*
  Product4 : Product
  Product6 : Product
  Selector : Selector  InputPortWidth=2  IndexOptions=Index vector (dialog)  Indices=1  OutputSizes=1
  Selector1 : Selector  InputPortWidth=2  IndexOptions=Index vector (dialog)  Indices=2  OutputSizes=1
  Selector2 : Selector  InputPortWidth=2  IndexOptions=Index vector (dialog)  Indices=1  OutputSizes=1
  Sum : Sum  Inputs=-+|
  Sum2 : Sum  Inputs=+--
  Terminator : Terminator
  Transpose1 : Math  Operator=transpose
  Vt_model : Outport
  H : Outport  Port=2
  F : Outport  Port=3
  G : Outport  Port=4
  wires:
  Gain/1 -> Mux/1
  Selector/1 -> 2-D Lookup Table R1/1, 2-D Lookup Table R0/1, 2-D Lookup Table V0/1, 2-D Lookup Table dV0/1, 2-D Lookup Table C1/1  "SOC"
  x/1 -> Probe/1, Selector/1, Selector1/1
  Math Function/1 -> Sum/1, Assignment/2
  2-D Lookup Table R1/1 -> Product4/2, Product/1  "R1"
  2-D Lookup Table C1/1 -> Product/2  "C1"
  Product2/1 -> Math Function/1
  Assignment/1 -> F/1
  Sum/1 -> Product4/1
  -Ts/1 -> Data Type Conversion Inherited/1, Data Type Conversion Inherited1/1, Gain/1, Product2/2
  Product4/1 -> Mux/2
  Mux/1 -> G/1
  2-D Lookup Table R0/1 -> Product6/1  "R0"
  Product6/1 -> Sum2/2
  Selector1/1 -> Sum2/3  "V1"
  current/1 -> Product6/2
  Mux1/1 -> Transpose1/1
  Transpose1/1 -> H/1
  Sum2/1 -> Vt_model/1
  2-D Lookup Table V0/1 -> Sum2/1  "V0"
  2-D Lookup Table dV0/1 -> Data Type Conversion Inherited2/1, Mux1/1  "dV0"
  Product/1 -> Product2/1  "tau1"
  Probe/1 -> Selector2/1
  Selector2/1 -> -Ts/1
  Data Type Conversion Inherited/1 -> Assignment/1
  Constant/1 -> Data Type Conversion Inherited/2
  Data Type Conversion Inherited1/1 -> Sum/2
  Constant1/1 -> Data Type Conversion Inherited1/2
  Data Type Conversion Inherited2/1 -> Mux1/2
  Constant4/1 -> Data Type Conversion Inherited2/2
  Temperature/1 -> Terminator/1
